simulink model "QPSKTx"  (R2017b)
settings: Solver=FixedStepDiscrete  StartTime=0.0  StopTime=inf  FixedStep=1/9.7656e+04  RelTol=1e-3  EnableMultiTasking=on
libraries: commdigbbndpm3 x1, commsdrhw_v2 x1
settings Model: Creator=Lab  LastModifiedBy=Lab
settings SolverCC: ConcurrentTasks=on  AutoInsertRateTranBlk=on  DecoupledContinuousIntegration=on

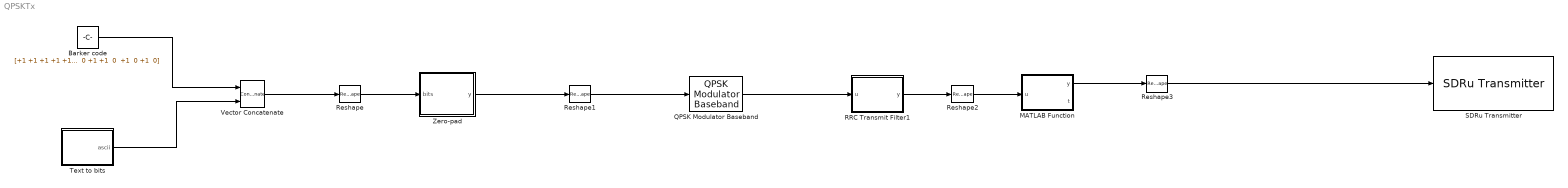
== system QPSKTx ==
  Barker code : Constant  Value="[+1 +1 +1 +1 +1 0  0 +1 +1  0  +1  0 +1  0 +1 +1 +1 +1 +1 0  0 +1 +1  0  +1  0 +1  0]"  VectorParams1D=off  SampleTime=-1
  MATLAB Function : MATLAB Function  TreatAsAtomicUnit=on
  QPSK Modulator Baseband : commdigbbndpm3/QPSK Modulator Baseband  InType=Bit  Enc=Gray  Ph=pi/4  outDtype=double  outWordLen=16  outUDDataType=sfix(16)  outFracLenMode=Best precision  outFracLen=15  outDataTypeStr=double  outLastDataTypeStr=double
  RRC Transmit Filter1 : MATLAB Function  TreatAsAtomicUnit=on
  Reshape{,1..3} (4 alike) : Reshape  OutputDimensionality=Column vector (2-D)
  SDRu Transmitter : commsdrhw_v2/SDRu Transmitter  SourceLibraryInfo="This block requires <a href=\"http://www.mathworks.com/hardware-support/usrp.html\">Communications System Toolbox Support Package for USRP Radio</a>"  rxtx=tx  platform=N200/N210/USRP2  USRP2_IP='192.168.10.8'  USRP_IP_X300='192.168.10.2'  USRP_IP_X310='192.168.10.2'  USRP_serialNumB200=''  USRP_serialNumB210=''  ChannelMapping=1  centerFrequency=20e6  centerFrequencySrc=Dialog  loOffset=0  loOffsetSrc=Dialog  PPSSource=Internal  clockSource=Internal  masterClkRateB200=32e6  masterClkRateB210=32e6  masterClkRateX300=200e6  masterClkRateX310=200e6  masterClkRateParam=100e6  gain=31  gainSrc=Dialog  decimInterp=256  decimInterpSrc=Dialog  TransportDataType=int16  USRP2_IP_NUM=[49 57 50 46 49 54 56 46 49 48 46 56]  frameLength=362  outputDatatype=Same as transport data type  overrunUnderrunPort=off  sampleTime=1  dboardInfo=|  HOST_DATA_PORT=30000  HOST_CONTROL_PORT=30001  USRP2_DATA_PORT=32769  USRP2_CONTROL_PORT=32768  bufferMode=Guaranteed contiguous buffer  EnableBurstMode=on  NumFramesInBurst=2  USRP_ID='192.168.10.8'
      | dbid: 0
      |           dbName: 'no db found'
      |          freqMin: 0
      |          freqMax: 0
      |          gainMin: 0
      |          gainMax: 0
      |     gainStepSize: 0
      settings: SourceProductName=Communications System Toolbox Support Package for USRP(R) Radio  SourceProductBaseCode=USRP
  "Text to bits " : MATLAB Function  TreatAsAtomicUnit=on
  Vector Concatenate : Concatenate
  "Zero-pad " : MATLAB Function  TreatAsAtomicUnit=on
  wires:
  Reshape2/1 -> MATLAB Function/1(u)
  Reshape/1 -> "Zero-pad "/1(bits)
  RRC Transmit Filter1/1(y) -> Reshape2/1
  Barker code/1 -> Vector Concatenate/1
  "Text to bits "/1(ascii) -> Vector Concatenate/2
  MATLAB Function/1(y) -> Reshape3/1
  Vector Concatenate/1 -> Reshape/1
  "Zero-pad "/1(y) -> Reshape1/1
  QPSK Modulator Baseband/1 -> RRC Transmit Filter1/1(u)
  Reshape1/1 -> QPSK Modulator Baseband/1
  Reshape3/1 -> SDRu Transmitter/1

== matlab function QPSKTx/RRC Transmit Filter1 ==
  data: u input; y output
function y = RRC(u)

rollOff = 0.6; 
span = 10; 
sps = 12; 

h = rcosdesign(rollOff, span, sps, 'sqrt'); 
symbs = upsample(u, sps); 
y = conv(symbs, h); 




end

== matlab function QPSKTx/Text to bits  ==
  data: ascii output

function ascii = fcn
    frame_length = 100; 
    txt = 'Hello World #0 Hello World #1 Hello World #2 Hello World #3';
%     txt = 'Why the fuck is this working? Why the fuck is working? '; 
    str = char(zeros(1, frame_length));
    
    % Pad message with char(1)'s to make the frame 100 long
    if length(txt) < frame_length 
        pad = 42*ones(1,frame_length-length(txt));
%         pad = randi([100 250], 1, frame_length-length(txt)); 
        tmp = double(txt); 
        tmp1 = [tmp pad]; 
        str = char(tmp1); 
        
    end
    
    
    
    symbols = zeros(1, length(str));
    bits =  zeros(length(str), 8); 
    ascii = zeros(1,8*length(str)); 
    
    
     
    
    symbols = double(char(str));
    bits = de2bi(symbols, 'left-msb', 8);
    
   
    ascii = reshape(bits', [1 8*size((bits),1)]);
    
    %% test with 00 01 10 11
%     txt=[0 0 0 1 1 0 1 1 0 0 0 1 1 0 1 1 0 0 0 1 1 0 1 1 0 0 0 1 1 0 1 1 0 0 0 1 1 0 1 1 0 0 0 1 1 0 1 1];
%        if length(txt) < frame_length 
%         pad = 42*zeros(1,frame_length-length(txt)); 
%         tmp1 = [txt pad]; 
%        end
%    ascii=tmp1;
%        
%         
   
end

== matlab function QPSKTx/MATLAB Function ==
  data: y output; t output; u input

% clc, clear, close
% 
% [signalPB, t] = exponential(); 
% % plot(t,real(y))
% 
% 
% 
% fs = 390625; 
% NFFT=2^11;      
% L=length(signalPB);         
% X= fftshift(fft(signalPB,NFFT));         
% Px=X.*conj(X)/(NFFT*L);      
% fVals=fs*(-NFFT/2:NFFT/2-1)/NFFT;        
% 
% 
% subplot(1,2,1)
% plot(fVals,10*log10(Px/max(Px)));    
% axis tight
% title('Power Spectral Density');         
% xlabel('Frequency (Hz)')         
% ylabel('Power (dB)');
% 
% 
% subplot(1,2,2)
% plot(real(signalPB))
% axis tight
% title('Passband signal')
% xlabel('Samples')
% ylabel('Amplitude')
% 


function [y,t] = exponential(u)
    N = 1024*3;

    y = complex(zeros(length(u)+N, 1)); 
    
    fs = 390625; 
    fc = 20e3;

    
    t = (0:1/fs:(N-1)/fs);
    
    tmp = exp(1i*2*pi*fc.*t');
  
   
    y = [u;  tmp;]; 
    
end

== matlab function QPSKTx/Zero-pad  ==
  data: bits input; y output
function y = fcn(bits)
%     len = length(bits); 
%     a = ceil(len/4);
%     padding=zeros(4*a-len, 1);
%     
%     
%     y = zeros(4*a,1); 
%     y = [bits; padding]; 
    
      y = bits; 
end
